simulink model "Scenario_3_v2"  (R2020b)
settings: Solver=ode1be  StartTime=0.0  StopTime=0.5  FixedStep=Ts  MaxStep=Ts/10  MinStep=Ts/40  RelTol=1e-3
values from neighbouring files (symbols this model uses):
  c0 = c0_zeb    (= 6.57988e-09)    [Scenario_17_parameters_v2.m]    (also in Scenario_1_parameters_v2.m; Scenario_2_parameters_v2.m; Scenario_3_parameters_v2.m)
  c0_hawk = 6.37282e-09    [Scenario_17_parameters_v2.m]    (also in Scenario_1_parameters_v2.m; Scenario_2_parameters_v2.m; Scenario_3_parameters_v2.m)
  c1 = c1_zeb    (= 9.15905e-09)    [Scenario_17_parameters_v2.m]    (also in Scenario_1_parameters_v2.m; Scenario_2_parameters_v2.m; Scenario_3_parameters_v2.m)
  c1_hawk = 8.76156e-09    [Scenario_17_parameters_v2.m]    (also in Scenario_1_parameters_v2.m; Scenario_2_parameters_v2.m; Scenario_3_parameters_v2.m)
  fg = 50    [Scenario_17_parameters_v2.m]    (also in Scenario_1_parameters_v2.m; Scenario_2_parameters_v2.m; Scenario_3_parameters_v2.m)
  G10gen = 0.90    (= 0.9)    [Scenario_3_parameters_v2.m]
  G12gen = 0.85    [Scenario_3_parameters_v2.m]
  G1gen = 0.4692    [Scenario_17_parameters_v2.m]    (also in Scenario_1_parameters_v2.m = 0.1; Scenario_2_parameters_v2.m = 0.298581; Scenario_3_parameters_v2.m = 0.65)
  G2gen = 0.80    (= 0.8)    [Scenario_1_parameters_v2.m]    (also in Scenario_2_parameters_v2.m = 0.7; Scenario_3_parameters_v2.m = 0.4)
  G3gen = 0.85    [Scenario_1_parameters_v2.m]    (also in Scenario_2_parameters_v2.m = 0.9; Scenario_3_parameters_v2.m = 0.6)
  G4gen = 0.65    [Scenario_3_parameters_v2.m]
  G5gen = 0.75    [Scenario_17_parameters_v2.m]    (also in Scenario_1_parameters_v2.m = 0.8; Scenario_2_parameters_v2.m = 0.8; Scenario_3_parameters_v2.m = 0.705)
  G6gen = 0.90    (= 0.9)    [Scenario_17_parameters_v2.m]    (also in Scenario_1_parameters_v2.m; Scenario_2_parameters_v2.m = 0.81797; Scenario_3_parameters_v2.m = 0.45)
  G7gen = 0.20    (= 0.2)    [Scenario_17_parameters_v2.m]    (also in Scenario_1_parameters_v2.m = 0.5227; Scenario_2_parameters_v2.m = 0.5098; Scenario_3_parameters_v2.m = 0.4)
  G8gen = 0.58    [Scenario_17_parameters_v2.m]    (also in Scenario_3_parameters_v2.m = 0.65)
  G9gen = 0.8833    [Scenario_17_parameters_v2.m]    (also in Scenario_3_parameters_v2.m = 0.9)
  Iovc = 1.2    [Scenario_17_parameters_v2.m]    (also in Scenario_1_parameters_v2.m; Scenario_2_parameters_v2.m; Scenario_3_parameters_v2.m)
  l0 = l0_zeb    (= 0.00368)    [Scenario_17_parameters_v2.m]    (also in Scenario_1_parameters_v2.m; Scenario_2_parameters_v2.m; Scenario_3_parameters_v2.m)
  l0_hawk = 0.00373    [Scenario_17_parameters_v2.m]    (also in Scenario_1_parameters_v2.m; Scenario_2_parameters_v2.m; Scenario_3_parameters_v2.m)
  l1 = l1_zeb    (= 0.00128)    [Scenario_17_parameters_v2.m]    (also in Scenario_1_parameters_v2.m; Scenario_2_parameters_v2.m; Scenario_3_parameters_v2.m)
  L10dem = 0.04    [Scenario_3_parameters_v2.m]
  L12dem = 0.01    [Scenario_17_parameters_v2.m]    (also in Scenario_3_parameters_v2.m = 0.02)
  L13dem = 0.01    [Scenario_3_parameters_v2.m]
  l1_hawk = 0.00133    [Scenario_17_parameters_v2.m]    (also in Scenario_1_parameters_v2.m; Scenario_2_parameters_v2.m; Scenario_3_parameters_v2.m)
  L1dem = 0.25    [Scenario_17_parameters_v2.m]    (also in Scenario_3_parameters_v2.m = 0.1)
  L3dem = 0.30    (= 0.3)    [Scenario_17_parameters_v2.m]    (also in Scenario_1_parameters_v2.m = 0.1; Scenario_2_parameters_v2.m = 0.1; Scenario_3_parameters_v2.m = 0.2)
  L5dem = 0.25    [Scenario_17_parameters_v2.m]    (also in Scenario_1_parameters_v2.m = 0.35; Scenario_2_parameters_v2.m = 0.35; Scenario_3_parameters_v2.m = 0.1)
  L6dem = 0.15    [Scenario_1_parameters_v2.m]    (also in Scenario_2_parameters_v2.m; Scenario_3_parameters_v2.m = 0.1)
  L7dem = 0.10    (= 0.1)    [Scenario_1_parameters_v2.m]    (also in Scenario_2_parameters_v2.m; Scenario_3_parameters_v2.m = 0.2)
  L9dem = 0.15    [Scenario_17_parameters_v2.m]    (also in Scenario_3_parameters_v2.m = 0.1)
  Pr = Sr*PF    (= 1600500000)    [Scenario_17_parameters_v2.m]    (also in Scenario_1_parameters_v2.m = 1472500000; Scenario_2_parameters_v2.m = 1805000000; Scenario_3_parameters_v2.m = 12740000000)
  Qr = sqrt(Sr^2 - Pr^2)    [Scenario_17_parameters_v2.m]    (also in Scenario_1_parameters_v2.m; Scenario_2_parameters_v2.m; Scenario_3_parameters_v2.m)
  r0 = r0_zeb    (= 0.39362)    [Scenario_17_parameters_v2.m]    (also in Scenario_1_parameters_v2.m; Scenario_2_parameters_v2.m; Scenario_3_parameters_v2.m)
  r0_hawk = 0.44587    [Scenario_17_parameters_v2.m]    (also in Scenario_1_parameters_v2.m; Scenario_2_parameters_v2.m; Scenario_3_parameters_v2.m)
  r1 = r1_zeb    (= 0.06862)    [Scenario_17_parameters_v2.m]    (also in Scenario_1_parameters_v2.m; Scenario_2_parameters_v2.m; Scenario_3_parameters_v2.m)
  r1_hawk = 0.12087    [Scenario_17_parameters_v2.m]    (also in Scenario_1_parameters_v2.m; Scenario_2_parameters_v2.m; Scenario_3_parameters_v2.m)
  Rtpu = Xtpu/40    (= 0.0025)    [Scenario_17_parameters_v2.m]    (also in Scenario_1_parameters_v2.m = 0.00375; Scenario_2_parameters_v2.m = 0.00375; Scenario_3_parameters_v2.m)
  S10non = 500e6    (= 500000000)    [Scenario_3_parameters_v2.m]
  S12non = 250e6    (= 250000000)    [Scenario_3_parameters_v2.m]
  S1non = 700e6    (= 700000000)    [Scenario_17_parameters_v2.m]    (also in Scenario_1_parameters_v2.m = 400000000; Scenario_2_parameters_v2.m = 400000000; Scenario_3_parameters_v2.m = 1000000000)
  S2non = 300e6    (= 300000000)    [Scenario_1_parameters_v2.m]    (also in Scenario_2_parameters_v2.m; Scenario_3_parameters_v2.m = 3000000000)
  S3non = 200e6    (= 200000000)    [Scenario_1_parameters_v2.m]    (also in Scenario_2_parameters_v2.m; Scenario_3_parameters_v2.m = 1000000000)
  S4non = 2000e6    (= 2000000000)    [Scenario_3_parameters_v2.m]
  S5non = 400e6    (= 400000000)    [Scenario_17_parameters_v2.m]    (also in Scenario_1_parameters_v2.m = 500000000; Scenario_2_parameters_v2.m = 500000000; Scenario_3_parameters_v2.m = 2000000000)
  S6non = 150e6    (= 150000000)    [Scenario_17_parameters_v2.m]    (also in Scenario_1_parameters_v2.m = 400000000; Scenario_2_parameters_v2.m = 400000000; Scenario_3_parameters_v2.m = 3000000000)
  S7non = 1500e6    (= 1500000000)    [Scenario_17_parameters_v2.m]    (also in Scenario_1_parameters_v2.m = 200000000; Scenario_2_parameters_v2.m = 200000000; Scenario_3_parameters_v2.m = 4000000000)
  S8non = 600e6    (= 600000000)    [Scenario_17_parameters_v2.m]    (also in Scenario_3_parameters_v2.m = 2000000000)
  S9non = 200e6    (= 200000000)    [Scenario_17_parameters_v2.m]    (also in Scenario_3_parameters_v2.m = 1500000000)
  tonvsc = 0    [Scenario_17_parameters_v2.m]    (also in Scenario_1_parameters_v2.m; Scenario_2_parameters_v2.m; Scenario_3_parameters_v2.m = 0.0001)
  Ts = 50e-6    (= 5e-05)    [Scenario_17_parameters_v2.m]    (also in Scenario_1_parameters_v2.m = 0.0002; Scenario_2_parameters_v2.m = 2e-05; Scenario_3_parameters_v2.m = 0.0001)
  Vhv = 220e3    (= 220000)    [Scenario_17_parameters_v2.m]    (also in Scenario_1_parameters_v2.m; Scenario_2_parameters_v2.m; Scenario_3_parameters_v2.m)
  Vmv = 22e3    (= 22000)    [Scenario_17_parameters_v2.m]    (also in Scenario_1_parameters_v2.m; Scenario_2_parameters_v2.m; Scenario_3_parameters_v2.m)
  w_pll = 2*pi*80    (= 502.654824574)    [Scenario_17_parameters_v2.m]    (also in Scenario_1_parameters_v2.m; Scenario_2_parameters_v2.m; Scenario_3_parameters_v2.m)
  wc1 = wsw1/10    (= 848.230016469)    [Scenario_17_parameters_v2.m]    (also in Scenario_1_parameters_v2.m; Scenario_2_parameters_v2.m; Scenario_3_parameters_v2.m)
  wdc1 = wc1/10    (= 84.8230016469)    [Scenario_17_parameters_v2.m]    (also in Scenario_1_parameters_v2.m; Scenario_2_parameters_v2.m; Scenario_3_parameters_v2.m)
  wpq1 = wc1/10    (= 84.8230016469)    [Scenario_17_parameters_v2.m]    (also in Scenario_1_parameters_v2.m; Scenario_2_parameters_v2.m; Scenario_3_parameters_v2.m)
  wsw1 = ksw1*2*pi*fg    (= 8482.30016469)    [Scenario_17_parameters_v2.m]    (also in Scenario_1_parameters_v2.m; Scenario_2_parameters_v2.m; Scenario_3_parameters_v2.m)
  Xtpu = 0.10    (= 0.1)    [Scenario_17_parameters_v2.m]    (also in Scenario_1_parameters_v2.m = 0.15; Scenario_2_parameters_v2.m = 0.15; Scenario_3_parameters_v2.m)
undefined symbols (not defined in the file or in its folder): D11, Delta
libraries: powerlib x428, simulink_extras x272, powerlib_meascontrol x194, pid_lib x105, simulink x60, eeTransforms x54, spsFirstOrderFilterLib x36, eePwmGeneratorTwoLevel x9
(part 8 of 40)

== system Scenario_3_v2/G6/VSC v2 ==
  note: If using different transformer connection,
      | compensate the delay in the modulation
  Pset : Inport
  Qset : Inport  Port=2
  Block : Step  Time=tonvsc  Before=1  After=0  SampleTime=0
  NOT : Logic  Operator=NOT  IconShape=distinctive  AllPortsSameDT=off  OutDataTypeStr=boolean
  Three-Phase Transformer (Two Windings) : powerlib/Elements/Three-Phase Transformer (Two Windings)  Winding1Connection=Yg  Winding2Connection=Delta (D11)  CoreType=Three single-phase transformers  SetSaturation=off  Hysteresis=off  DataFile='hysteresis'  SetInitialFlux=off  Measurements=None  UNITS=pu  NominalPower=[Pconv , fg ]  Winding1=[Vhv, Rtpu/2, Xtpu/2]  Winding2=[Vmv, Rtpu/2, Xtpu/2]  Rm=5000  Lm=5000  L0=0.5  Saturation=[ 0,0 ; 0.0024,1.2 ; 1.0,1.52 ]  InitialFluxes=[ 0.8 , -0.8 , 0.7 ]  BreakLoop=off  DiscreteSolver=Trapezoidal iterative  DataType=off  TransfoNumber=1
  Three-Phase Breaker : powerlib/Elements/Three-Phase Breaker  InitialState=open  SwitchA=on  SwitchB=on  SwitchC=on  SwitchTimes="[1/60  5/60]"  External=on  BreakerResistance=0.001  SnubberResistance=1e7  SnubberCapacitance=inf  Measurements=None
  VI measurement : Subsystem
      settings: PortSchema="{\"entries\":[{\"content\":{\"sides\":[{\"content\":{\"connectorIds\":[\"LConn1\",\"LConn2\",\"LConn3\"]},\"type\":\"ConnectorPlacement.EquallySpacedRectSide\",\"uuid\":\"d0d5b0b8-afec-4f90-9eba-536a06b10059\"},{\"content\":{\"connectorIds\":[\"RConn1\",\"RConn2\",\"RConn3\"],\"side\":\"RIGHT\"},\"type\":\"ConnectorPlacement.EquallySpacedRectSide\",\"uuid\":\"adc1b68d-6172-4507-b54b-9373921355a1\"},{\"content\":{\"connectorIds\":[\"Out1\",\"Out2\"],\"side\":\"TOP\"},\"type\":\"ConnectorPlacement.EquallySpacedRectSide\",\"uuid\":\"8c5adf07-e95b-4907-94c3-1b2a47d47f40\"}]},\"type\":\"ConnectorPlacement.EquallySpacedConnector\",\"uuid\":\"87d0b20f-8f85-4790-a611-3415e642a83a\"}],\"packageUris\":[\"http://schema.mathworks.com/mf0/Connector/R2020b\"],\"version\":\"1.0\"}"
  VSC Control : Subsystem
      settings: PortSchema="{\"entries\":[{\"content\":{\"sides\":[{\"content\":{\"connectorIds\":[\"In1\",\"In2\",\"In3\",\"In4\",\"In5\",\"In6\"]},\"type\":\"ConnectorPlacement.EquallySpacedRectSide\",\"uuid\":\"cada8d9e-53e0-4197-9386-6c7b6ea13844\"},{\"content\":{\"connectorIds\":[\"Out1\"],\"side\":\"RIGHT\"},\"type\":\"ConnectorPlacement.EquallySpacedRectSide\",\"uuid\":\"f237b52a-0d77-45c0-937d-32cafba1283e\"},{\"content\":{\"connectorIds\":[\"Out2\"],\"side\":\"TOP\"},\"type\":\"ConnectorPlacement.EquallySpacedRectSide\",\"uuid\":\"e6f268b5-5f09-49a6-9529-b1aeebd5f021\"}]},\"type\":\"ConnectorPlacement.EquallySpacedConnector\",\"uuid\":\"4d1d2957-2eb9-4111-8c87-957e800b2b0b\"}],\"packageUris\":[\"http://schema.mathworks.com/mf0/Connector/R2020b\"],\"version\":\"1.0\"}"
  VSC Model : Subsystem  Variant=on  VariantControlMode=label  LabelModeActiveChoice=EMT_AVG
      settings: PortSchema="{\"entries\":[{\"content\":{\"sides\":[{\"content\":{\"connectorIds\":[\"LConn1\",\"LConn2\",\"LConn3\"]},\"type\":\"ConnectorPlacement.EquallySpacedRectSide\",\"uuid\":\"96043b84-a665-4cb2-a938-d6633d7ee474\"},{\"content\":{\"connectorIds\":[\"In1\"],\"side\":\"RIGHT\"},\"type\":\"ConnectorPlacement.EquallySpacedRectSide\",\"uuid\":\"064d463f-c23a-42ac-89ce-8dea3d446214\"},{\"content\":{\"connectorIds\":[],\"side\":\"TOP\"},\"type\":\"ConnectorPlacement.EquallySpacedRectSide\",\"uuid\":\"95ef669c-c6ed-44c3-8b69-447906728b6d\"}]},\"type\":\"ConnectorPlacement.EquallySpacedConnector\",\"uuid\":\"ea66db09-64d7-4d7e-ba7b-d769c56e2dbd\"}],\"packageUris\":[\"http://schema.mathworks.com/mf0/Connector/19700101\"],\"version\":\"1.0\"}"
  output signals : Subsystem
  A : PMIOPort  Side=Left
  B : PMIOPort  Port=2  Side=Left
  C : PMIOPort  Port=3  Side=Left
  m : Outport
  wires:
  NOT/1 -> Three-Phase Breaker/1
  VSC Control/1(Ref) -> VSC Model/1(Ref)
  [Is] -> VSC Control/3(Iabc)
  Block/1 -> NOT/1, VSC Control/1(Block)
  [Vs] -> output signals/1(Vs)
  [Is] -> output signals/2(Is)
  VSC Control/2(m) -> output signals/3(control)
  output signals/1(m) -> m/1
  VI measurement/1(Vs) -> [Vs]
  VI measurement/2(Is) -> [Is]
  Qset/1 -> VSC Control/5(Qset)
  [Vs] -> VSC Control/2(Vabc)
  ? -> VSC Control/6(Edc)
  Pset/1 -> VSC Control/4(Pset)
  connections:
  Three-Phase Transformer (Two Windings)/LConn3 -- Three-Phase Breaker/LConn3
  Three-Phase Transformer (Two Windings)/LConn2 -- Three-Phase Breaker/LConn2
  Three-Phase Transformer (Two Windings)/LConn1 -- Three-Phase Breaker/LConn1
  Three-Phase Transformer (Two Windings)/RConn3 -- VSC Model/LConn3
  Three-Phase Transformer (Two Windings)/RConn2 -- VSC Model/LConn2
  Three-Phase Transformer (Two Windings)/RConn1 -- VSC Model/LConn1
  VI measurement/RConn1 -- A/RConn1
  VI measurement/RConn2 -- B/RConn1
  VI measurement/RConn3 -- C/RConn1
  VI measurement/LConn1 -- Three-Phase Breaker/RConn1
  VI measurement/LConn2 -- Three-Phase Breaker/RConn2
  VI measurement/LConn3 -- Three-Phase Breaker/RConn3

== system Scenario_3_v2/G7/VSC v2 ==
  note: If using different transformer connection,
      | compensate the delay in the modulation
  Pset : Inport
  Qset : Inport  Port=2
  Block : Step  Time=tonvsc  Before=1  After=0  SampleTime=0
  NOT : Logic  Operator=NOT  IconShape=distinctive  AllPortsSameDT=off  OutDataTypeStr=boolean
  Three-Phase Transformer (Two Windings) : powerlib/Elements/Three-Phase Transformer (Two Windings)  Winding1Connection=Yg  Winding2Connection=Delta (D11)  CoreType=Three single-phase transformers  SetSaturation=off  Hysteresis=off  DataFile='hysteresis'  SetInitialFlux=off  Measurements=None  UNITS=pu  NominalPower=[Pconv , fg ]  Winding1=[Vhv, Rtpu/2, Xtpu/2]  Winding2=[Vmv, Rtpu/2, Xtpu/2]  Rm=5000  Lm=5000  L0=0.5  Saturation=[ 0,0 ; 0.0024,1.2 ; 1.0,1.52 ]  InitialFluxes=[ 0.8 , -0.8 , 0.7 ]  BreakLoop=off  DiscreteSolver=Trapezoidal iterative  DataType=off  TransfoNumber=1
  Three-Phase Breaker : powerlib/Elements/Three-Phase Breaker  InitialState=open  SwitchA=on  SwitchB=on  SwitchC=on  SwitchTimes="[1/60  5/60]"  External=on  BreakerResistance=0.001  SnubberResistance=1e7  SnubberCapacitance=inf  Measurements=None
  VI measurement : Subsystem
      settings: PortSchema="{\"entries\":[{\"content\":{\"sides\":[{\"content\":{\"connectorIds\":[\"LConn1\",\"LConn2\",\"LConn3\"]},\"type\":\"ConnectorPlacement.EquallySpacedRectSide\",\"uuid\":\"d0d5b0b8-afec-4f90-9eba-536a06b10059\"},{\"content\":{\"connectorIds\":[\"RConn1\",\"RConn2\",\"RConn3\"],\"side\":\"RIGHT\"},\"type\":\"ConnectorPlacement.EquallySpacedRectSide\",\"uuid\":\"adc1b68d-6172-4507-b54b-9373921355a1\"},{\"content\":{\"connectorIds\":[\"Out1\",\"Out2\"],\"side\":\"TOP\"},\"type\":\"ConnectorPlacement.EquallySpacedRectSide\",\"uuid\":\"8c5adf07-e95b-4907-94c3-1b2a47d47f40\"}]},\"type\":\"ConnectorPlacement.EquallySpacedConnector\",\"uuid\":\"87d0b20f-8f85-4790-a611-3415e642a83a\"}],\"packageUris\":[\"http://schema.mathworks.com/mf0/Connector/R2020b\"],\"version\":\"1.0\"}"
  VSC Control : Subsystem
      settings: PortSchema="{\"entries\":[{\"content\":{\"sides\":[{\"content\":{\"connectorIds\":[\"In1\",\"In2\",\"In3\",\"In4\",\"In5\",\"In6\"]},\"type\":\"ConnectorPlacement.EquallySpacedRectSide\",\"uuid\":\"cada8d9e-53e0-4197-9386-6c7b6ea13844\"},{\"content\":{\"connectorIds\":[\"Out1\"],\"side\":\"RIGHT\"},\"type\":\"ConnectorPlacement.EquallySpacedRectSide\",\"uuid\":\"f237b52a-0d77-45c0-937d-32cafba1283e\"},{\"content\":{\"connectorIds\":[\"Out2\"],\"side\":\"TOP\"},\"type\":\"ConnectorPlacement.EquallySpacedRectSide\",\"uuid\":\"e6f268b5-5f09-49a6-9529-b1aeebd5f021\"}]},\"type\":\"ConnectorPlacement.EquallySpacedConnector\",\"uuid\":\"4d1d2957-2eb9-4111-8c87-957e800b2b0b\"}],\"packageUris\":[\"http://schema.mathworks.com/mf0/Connector/R2020b\"],\"version\":\"1.0\"}"
  VSC Model : Subsystem  Variant=on  VariantControlMode=label  LabelModeActiveChoice=EMT_AVG
      settings: PortSchema="{\"entries\":[{\"content\":{\"sides\":[{\"content\":{\"connectorIds\":[\"LConn1\",\"LConn2\",\"LConn3\"]},\"type\":\"ConnectorPlacement.EquallySpacedRectSide\",\"uuid\":\"96043b84-a665-4cb2-a938-d6633d7ee474\"},{\"content\":{\"connectorIds\":[\"In1\"],\"side\":\"RIGHT\"},\"type\":\"ConnectorPlacement.EquallySpacedRectSide\",\"uuid\":\"064d463f-c23a-42ac-89ce-8dea3d446214\"},{\"content\":{\"connectorIds\":[],\"side\":\"TOP\"},\"type\":\"ConnectorPlacement.EquallySpacedRectSide\",\"uuid\":\"95ef669c-c6ed-44c3-8b69-447906728b6d\"}]},\"type\":\"ConnectorPlacement.EquallySpacedConnector\",\"uuid\":\"ea66db09-64d7-4d7e-ba7b-d769c56e2dbd\"}],\"packageUris\":[\"http://schema.mathworks.com/mf0/Connector/19700101\"],\"version\":\"1.0\"}"
  output signals : Subsystem
  A : PMIOPort  Side=Left
  B : PMIOPort  Port=2  Side=Left
  C : PMIOPort  Port=3  Side=Left
  m : Outport
  wires:
  NOT/1 -> Three-Phase Breaker/1
  VSC Control/1(Ref) -> VSC Model/1(Ref)
  [Is] -> VSC Control/3(Iabc)
  Block/1 -> NOT/1, VSC Control/1(Block)
  [Vs] -> output signals/1(Vs)
  [Is] -> output signals/2(Is)
  VSC Control/2(m) -> output signals/3(control)
  output signals/1(m) -> m/1
  VI measurement/1(Vs) -> [Vs]
  VI measurement/2(Is) -> [Is]
  Qset/1 -> VSC Control/5(Qset)
  [Vs] -> VSC Control/2(Vabc)
  ? -> VSC Control/6(Edc)
  Pset/1 -> VSC Control/4(Pset)
  connections:
  Three-Phase Transformer (Two Windings)/LConn3 -- Three-Phase Breaker/LConn3
  Three-Phase Transformer (Two Windings)/LConn2 -- Three-Phase Breaker/LConn2
  Three-Phase Transformer (Two Windings)/LConn1 -- Three-Phase Breaker/LConn1
  Three-Phase Transformer (Two Windings)/RConn3 -- VSC Model/LConn3
  Three-Phase Transformer (Two Windings)/RConn2 -- VSC Model/LConn2
  Three-Phase Transformer (Two Windings)/RConn1 -- VSC Model/LConn1
  VI measurement/RConn1 -- A/RConn1
  VI measurement/RConn2 -- B/RConn1
  VI measurement/RConn3 -- C/RConn1
  VI measurement/LConn1 -- Three-Phase Breaker/RConn1
  VI measurement/LConn2 -- Three-Phase Breaker/RConn2
  VI measurement/LConn3 -- Three-Phase Breaker/RConn3

== system Scenario_3_v2/G9/VSC v2 ==
  note: If using different transformer connection,
      | compensate the delay in the modulation
  Pset : Inport
  Qset : Inport  Port=2
  Block : Step  Time=tonvsc  Before=1  After=0  SampleTime=0
  NOT : Logic  Operator=NOT  IconShape=distinctive  AllPortsSameDT=off  OutDataTypeStr=boolean
  Three-Phase Transformer (Two Windings) : powerlib/Elements/Three-Phase Transformer (Two Windings)  Winding1Connection=Yg  Winding2Connection=Delta (D11)  CoreType=Three single-phase transformers  SetSaturation=off  Hysteresis=off  DataFile='hysteresis'  SetInitialFlux=off  Measurements=None  UNITS=pu  NominalPower=[Pconv , fg ]  Winding1=[Vhv, Rtpu/2, Xtpu/2]  Winding2=[Vmv, Rtpu/2, Xtpu/2]  Rm=5000  Lm=5000  L0=0.5  Saturation=[ 0,0 ; 0.0024,1.2 ; 1.0,1.52 ]  InitialFluxes=[ 0.8 , -0.8 , 0.7 ]  BreakLoop=off  DiscreteSolver=Trapezoidal iterative  DataType=off  TransfoNumber=1
  Three-Phase Breaker : powerlib/Elements/Three-Phase Breaker  InitialState=open  SwitchA=on  SwitchB=on  SwitchC=on  SwitchTimes="[1/60  5/60]"  External=on  BreakerResistance=0.001  SnubberResistance=1e7  SnubberCapacitance=inf  Measurements=None
  VI measurement : Subsystem
      settings: PortSchema="{\"entries\":[{\"content\":{\"sides\":[{\"content\":{\"connectorIds\":[\"LConn1\",\"LConn2\",\"LConn3\"]},\"type\":\"ConnectorPlacement.EquallySpacedRectSide\",\"uuid\":\"d0d5b0b8-afec-4f90-9eba-536a06b10059\"},{\"content\":{\"connectorIds\":[\"RConn1\",\"RConn2\",\"RConn3\"],\"side\":\"RIGHT\"},\"type\":\"ConnectorPlacement.EquallySpacedRectSide\",\"uuid\":\"adc1b68d-6172-4507-b54b-9373921355a1\"},{\"content\":{\"connectorIds\":[\"Out1\",\"Out2\"],\"side\":\"TOP\"},\"type\":\"ConnectorPlacement.EquallySpacedRectSide\",\"uuid\":\"8c5adf07-e95b-4907-94c3-1b2a47d47f40\"}]},\"type\":\"ConnectorPlacement.EquallySpacedConnector\",\"uuid\":\"87d0b20f-8f85-4790-a611-3415e642a83a\"}],\"packageUris\":[\"http://schema.mathworks.com/mf0/Connector/R2020b\"],\"version\":\"1.0\"}"
  VSC Control : Subsystem
      settings: PortSchema="{\"entries\":[{\"content\":{\"sides\":[{\"content\":{\"connectorIds\":[\"In1\",\"In2\",\"In3\",\"In4\",\"In5\",\"In6\"]},\"type\":\"ConnectorPlacement.EquallySpacedRectSide\",\"uuid\":\"cada8d9e-53e0-4197-9386-6c7b6ea13844\"},{\"content\":{\"connectorIds\":[\"Out1\"],\"side\":\"RIGHT\"},\"type\":\"ConnectorPlacement.EquallySpacedRectSide\",\"uuid\":\"f237b52a-0d77-45c0-937d-32cafba1283e\"},{\"content\":{\"connectorIds\":[\"Out2\"],\"side\":\"TOP\"},\"type\":\"ConnectorPlacement.EquallySpacedRectSide\",\"uuid\":\"e6f268b5-5f09-49a6-9529-b1aeebd5f021\"}]},\"type\":\"ConnectorPlacement.EquallySpacedConnector\",\"uuid\":\"4d1d2957-2eb9-4111-8c87-957e800b2b0b\"}],\"packageUris\":[\"http://schema.mathworks.com/mf0/Connector/R2020b\"],\"version\":\"1.0\"}"
  VSC Model : Subsystem  Variant=on  VariantControlMode=label  LabelModeActiveChoice=EMT_AVG
      settings: PortSchema="{\"entries\":[{\"content\":{\"sides\":[{\"content\":{\"connectorIds\":[\"LConn1\",\"LConn2\",\"LConn3\"]},\"type\":\"ConnectorPlacement.EquallySpacedRectSide\",\"uuid\":\"96043b84-a665-4cb2-a938-d6633d7ee474\"},{\"content\":{\"connectorIds\":[\"In1\"],\"side\":\"RIGHT\"},\"type\":\"ConnectorPlacement.EquallySpacedRectSide\",\"uuid\":\"064d463f-c23a-42ac-89ce-8dea3d446214\"},{\"content\":{\"connectorIds\":[],\"side\":\"TOP\"},\"type\":\"ConnectorPlacement.EquallySpacedRectSide\",\"uuid\":\"95ef669c-c6ed-44c3-8b69-447906728b6d\"}]},\"type\":\"ConnectorPlacement.EquallySpacedConnector\",\"uuid\":\"ea66db09-64d7-4d7e-ba7b-d769c56e2dbd\"}],\"packageUris\":[\"http://schema.mathworks.com/mf0/Connector/19700101\"],\"version\":\"1.0\"}"
  output signals : Subsystem
  A : PMIOPort  Side=Left
  B : PMIOPort  Port=2  Side=Left
  C : PMIOPort  Port=3  Side=Left
  m : Outport
  wires:
  NOT/1 -> Three-Phase Breaker/1
  VSC Control/1(Ref) -> VSC Model/1(Ref)
  [Is] -> VSC Control/3(Iabc)
  Block/1 -> NOT/1, VSC Control/1(Block)
  [Vs] -> output signals/1(Vs)
  [Is] -> output signals/2(Is)
  VSC Control/2(m) -> output signals/3(control)
  output signals/1(m) -> m/1
  VI measurement/1(Vs) -> [Vs]
  VI measurement/2(Is) -> [Is]
  Qset/1 -> VSC Control/5(Qset)
  [Vs] -> VSC Control/2(Vabc)
  ? -> VSC Control/6(Edc)
  Pset/1 -> VSC Control/4(Pset)
  connections:
  Three-Phase Transformer (Two Windings)/LConn3 -- Three-Phase Breaker/LConn3
  Three-Phase Transformer (Two Windings)/LConn2 -- Three-Phase Breaker/LConn2
  Three-Phase Transformer (Two Windings)/LConn1 -- Three-Phase Breaker/LConn1
  Three-Phase Transformer (Two Windings)/RConn3 -- VSC Model/LConn3
  Three-Phase Transformer (Two Windings)/RConn2 -- VSC Model/LConn2
  Three-Phase Transformer (Two Windings)/RConn1 -- VSC Model/LConn1
  VI measurement/RConn1 -- A/RConn1
  VI measurement/RConn2 -- B/RConn1
  VI measurement/RConn3 -- C/RConn1
  VI measurement/LConn1 -- Three-Phase Breaker/RConn1
  VI measurement/LConn2 -- Three-Phase Breaker/RConn2
  VI measurement/LConn3 -- Three-Phase Breaker/RConn3

== system Scenario_3_v2/HVDC/DC-link ==
  note: Diagram of the DC link
  note: The DC link dynamics is calculated in state-space intead of simulated using electric elements to allow both EMT and Phasor use the same block in the simulations
  note: | vdc1 |
      | x = | vdc2 |
      | | idc |
  note: The model states are the DC voltages of the two terminals and the DC current:
  note: idc1
  note: idc2
  note: The model outputs are the DC voltages of the two terminals
  idc1 : Inport
  idc2 : Inport  Port=2
  C1 : powerlib/Elements/Series RLC Branch  Commented=on  LConnTagsString=__new0  RConnTagsString=__new0  BranchType=C  Resistance=R  Inductance=1e-3  SetiL0=off  InitialCurrent=0  Capacitance=1  Setx0=off  InitialVoltage=Vdc0  Measurements=None
  C2 : powerlib/Elements/Series RLC Branch  Commented=on  LConnTagsString=__new0  RConnTagsString=__new0  BranchType=C  Resistance=R  Inductance=1e-3  SetiL0=off  InitialCurrent=0  Capacitance=1  Setx0=off  InitialVoltage=Vdc0  Measurements=None
  Demux : Demux  Outputs=2
  Mux : Mux  Inputs=2
  RL : powerlib/Elements/Series RLC Branch  Commented=on  LConnTagsString=__new0  RConnTagsString=__new0  BranchType=RL  Resistance=1  Inductance=1  SetiL0=off  InitialCurrent=0  Capacitance=1e-6  Setx0=off  InitialVoltage=0  Measurements=None
  State-Space1 : StateSpace  A=[0 0 -1/C1 ; 0 0 1/C2 ; 1/L -1/L -R/L]  B=[1/C1 0 ; 0 1/C2; 0 0]  C=[1 0 0; 0 1 0]  D=[0 0; 0 0]  InitialCondition=[v1dc0; v2dc0; idc0]
  vdc1 : Outport
  vdc2 : Outport  Port=2
  wires:
  ? -> ?
  ? -> ?
  Mux/1 -> State-Space1/1
  idc1/1 -> Mux/1
  idc2/1 -> Mux/2
  State-Space1/1 -> Demux/1
  Demux/1 -> vdc1/1
  Demux/2 -> vdc2/1
  connections:
  C1/LConn1 -- RL/LConn1
  C2/LConn1 -- RL/RConn1

== system Scenario_3_v2/HVDC/VSC1 v2 ==
  note: If using different transformer connection,
      | compensate the delay in the modulation
  Pset : Inport
  Qset : Inport  Port=2
  Block : Step  Time=tonvsc  Before=1  After=0  SampleTime=0
  NOT : Logic  Operator=NOT  IconShape=distinctive  AllPortsSameDT=off  OutDataTypeStr=boolean
  Three-Phase Transformer (Two Windings) : powerlib/Elements/Three-Phase Transformer (Two Windings)  Winding1Connection=Yg  Winding2Connection=Delta (D11)  CoreType=Three single-phase transformers  SetSaturation=off  Hysteresis=off  DataFile='hysteresis'  SetInitialFlux=off  Measurements=None  UNITS=pu  NominalPower=[Pconv , fg ]  Winding1=[Vhv, Rtpu/2, Xtpu/2]  Winding2=[Vmv, Rtpu/2, Xtpu/2]  Rm=5000  Lm=5000  L0=0.5  Saturation=[ 0,0 ; 0.0024,1.2 ; 1.0,1.52 ]  InitialFluxes=[ 0.8 , -0.8 , 0.7 ]  BreakLoop=off  DiscreteSolver=Trapezoidal iterative  DataType=off  TransfoNumber=1
  Three-Phase Breaker : powerlib/Elements/Three-Phase Breaker  InitialState=open  SwitchA=on  SwitchB=on  SwitchC=on  SwitchTimes="[1/60  5/60]"  External=on  BreakerResistance=0.001  SnubberResistance=1e7  SnubberCapacitance=inf  Measurements=None
  VI measurement : Subsystem
      settings: PortSchema="{\"entries\":[{\"content\":{\"sides\":[{\"content\":{\"connectorIds\":[\"LConn1\",\"LConn2\",\"LConn3\"]},\"type\":\"ConnectorPlacement.EquallySpacedRectSide\",\"uuid\":\"d0d5b0b8-afec-4f90-9eba-536a06b10059\"},{\"content\":{\"connectorIds\":[\"RConn1\",\"RConn2\",\"RConn3\"],\"side\":\"RIGHT\"},\"type\":\"ConnectorPlacement.EquallySpacedRectSide\",\"uuid\":\"adc1b68d-6172-4507-b54b-9373921355a1\"},{\"content\":{\"connectorIds\":[\"Out1\",\"Out2\"],\"side\":\"TOP\"},\"type\":\"ConnectorPlacement.EquallySpacedRectSide\",\"uuid\":\"8c5adf07-e95b-4907-94c3-1b2a47d47f40\"}]},\"type\":\"ConnectorPlacement.EquallySpacedConnector\",\"uuid\":\"87d0b20f-8f85-4790-a611-3415e642a83a\"}],\"packageUris\":[\"http://schema.mathworks.com/mf0/Connector/R2020b\"],\"version\":\"1.0\"}"
  VSC Control : Subsystem
      settings: PortSchema="{\"entries\":[{\"content\":{\"sides\":[{\"content\":{\"connectorIds\":[\"In1\",\"In2\",\"In3\",\"In4\",\"In5\"]},\"type\":\"ConnectorPlacement.EquallySpacedRectSide\",\"uuid\":\"cada8d9e-53e0-4197-9386-6c7b6ea13844\"},{\"content\":{\"connectorIds\":[\"Out1\"],\"side\":\"RIGHT\"},\"type\":\"ConnectorPlacement.EquallySpacedRectSide\",\"uuid\":\"f237b52a-0d77-45c0-937d-32cafba1283e\"},{\"content\":{\"connectorIds\":[\"Out2\"],\"side\":\"TOP\"},\"type\":\"ConnectorPlacement.EquallySpacedRectSide\",\"uuid\":\"e6f268b5-5f09-49a6-9529-b1aeebd5f021\"}]},\"type\":\"ConnectorPlacement.EquallySpacedConnector\",\"uuid\":\"4d1d2957-2eb9-4111-8c87-957e800b2b0b\"}],\"packageUris\":[\"http://schema.mathworks.com/mf0/Connector/19700101\"],\"version\":\"1.0\"}"
  VSC Model : Subsystem  Variant=on  VariantControlMode=label  LabelModeActiveChoice=EMT_AVG
      settings: PortSchema="{\"entries\":[{\"content\":{\"sides\":[{\"content\":{\"connectorIds\":[\"LConn1\",\"LConn2\",\"LConn3\"]},\"type\":\"ConnectorPlacement.EquallySpacedRectSide\",\"uuid\":\"96043b84-a665-4cb2-a938-d6633d7ee474\"},{\"content\":{\"connectorIds\":[\"In1\"],\"side\":\"RIGHT\"},\"type\":\"ConnectorPlacement.EquallySpacedRectSide\",\"uuid\":\"064d463f-c23a-42ac-89ce-8dea3d446214\"},{\"content\":{\"connectorIds\":[],\"side\":\"TOP\"},\"type\":\"ConnectorPlacement.EquallySpacedRectSide\",\"uuid\":\"95ef669c-c6ed-44c3-8b69-447906728b6d\"}]},\"type\":\"ConnectorPlacement.EquallySpacedConnector\",\"uuid\":\"ea66db09-64d7-4d7e-ba7b-d769c56e2dbd\"}],\"packageUris\":[\"http://schema.mathworks.com/mf0/Connector/19700101\"],\"version\":\"1.0\"}"
  output signals : Subsystem
  A : PMIOPort  Side=Left
  B : PMIOPort  Port=2  Side=Left
  C : PMIOPort  Port=3  Side=Left
  m : Outport
  wires:
  NOT/1 -> Three-Phase Breaker/1
  VSC Control/1(Ref) -> VSC Model/1(Ref)
  [Is] -> VSC Control/3(Iabc)
  Block/1 -> NOT/1, VSC Control/1(Block)
  [Vs] -> output signals/1(Vs)
  [Is] -> output signals/2(Is)
  VSC Control/2(m) -> output signals/3(control)
  output signals/1(m) -> m/1
  VI measurement/1(Vs) -> [Vs]
  VI measurement/2(Is) -> [Is]
  Qset/1 -> VSC Control/5(Qset)
  Pset/1 -> VSC Control/4(Pset)
  [Vs] -> VSC Control/2(Vabc)
  connections:
  Three-Phase Transformer (Two Windings)/LConn3 -- Three-Phase Breaker/LConn3
  Three-Phase Transformer (Two Windings)/LConn2 -- Three-Phase Breaker/LConn2
  Three-Phase Transformer (Two Windings)/LConn1 -- Three-Phase Breaker/LConn1
  Three-Phase Transformer (Two Windings)/RConn3 -- VSC Model/LConn3
  Three-Phase Transformer (Two Windings)/RConn2 -- VSC Model/LConn2
  Three-Phase Transformer (Two Windings)/RConn1 -- VSC Model/LConn1
  VI measurement/RConn1 -- A/RConn1
  VI measurement/RConn2 -- B/RConn1
  VI measurement/RConn3 -- C/RConn1
  VI measurement/LConn1 -- Three-Phase Breaker/RConn1
  VI measurement/LConn2 -- Three-Phase Breaker/RConn2
  VI measurement/LConn3 -- Three-Phase Breaker/RConn3

== system Scenario_3_v2/HVDC/VSC2 v2 ==
  note: If using different transformer connection,
      | compensate the delay in the modulation
  Qset : Inport
  Edc : Inport  Port=2
  Block : Step  Time=tonvsc  Before=1  After=0  SampleTime=0
  NOT : Logic  Operator=NOT  IconShape=distinctive  AllPortsSameDT=off  OutDataTypeStr=boolean
  Three-Phase Transformer (Two Windings) : powerlib/Elements/Three-Phase Transformer (Two Windings)  Winding1Connection=Yg  Winding2Connection=Delta (D11)  CoreType=Three single-phase transformers  SetSaturation=off  Hysteresis=off  DataFile='hysteresis'  SetInitialFlux=off  Measurements=None  UNITS=pu  NominalPower=[Pconv , fg ]  Winding1=[Vhv, Rtpu/2, Xtpu/2]  Winding2=[Vmv, Rtpu/2, Xtpu/2]  Rm=5000  Lm=5000  L0=0.5  Saturation=[ 0,0 ; 0.0024,1.2 ; 1.0,1.52 ]  InitialFluxes=[ 0.8 , -0.8 , 0.7 ]  BreakLoop=off  DiscreteSolver=Trapezoidal iterative  DataType=off  TransfoNumber=1
  Three-Phase Breaker : powerlib/Elements/Three-Phase Breaker  InitialState=open  SwitchA=on  SwitchB=on  SwitchC=on  SwitchTimes="[1/60  5/60]"  External=on  BreakerResistance=0.001  SnubberResistance=1e7  SnubberCapacitance=inf  Measurements=None
  VI measurement : Subsystem
      settings: PortSchema="{\"entries\":[{\"content\":{\"sides\":[{\"content\":{\"connectorIds\":[\"LConn1\",\"LConn2\",\"LConn3\"]},\"type\":\"ConnectorPlacement.EquallySpacedRectSide\",\"uuid\":\"d0d5b0b8-afec-4f90-9eba-536a06b10059\"},{\"content\":{\"connectorIds\":[\"RConn1\",\"RConn2\",\"RConn3\"],\"side\":\"RIGHT\"},\"type\":\"ConnectorPlacement.EquallySpacedRectSide\",\"uuid\":\"adc1b68d-6172-4507-b54b-9373921355a1\"},{\"content\":{\"connectorIds\":[\"Out1\",\"Out2\"],\"side\":\"TOP\"},\"type\":\"ConnectorPlacement.EquallySpacedRectSide\",\"uuid\":\"8c5adf07-e95b-4907-94c3-1b2a47d47f40\"}]},\"type\":\"ConnectorPlacement.EquallySpacedConnector\",\"uuid\":\"87d0b20f-8f85-4790-a611-3415e642a83a\"}],\"packageUris\":[\"http://schema.mathworks.com/mf0/Connector/R2020b\"],\"version\":\"1.0\"}"
  VSC Control : Subsystem
      settings: PortSchema="{\"entries\":[{\"content\":{\"sides\":[{\"content\":{\"connectorIds\":[\"In1\",\"In2\",\"In3\",\"In4\",\"In5\",\"In6\"]},\"type\":\"ConnectorPlacement.EquallySpacedRectSide\",\"uuid\":\"cada8d9e-53e0-4197-9386-6c7b6ea13844\"},{\"content\":{\"connectorIds\":[\"Out1\"],\"side\":\"RIGHT\"},\"type\":\"ConnectorPlacement.EquallySpacedRectSide\",\"uuid\":\"f237b52a-0d77-45c0-937d-32cafba1283e\"},{\"content\":{\"connectorIds\":[\"Out2\"],\"side\":\"TOP\"},\"type\":\"ConnectorPlacement.EquallySpacedRectSide\",\"uuid\":\"e6f268b5-5f09-49a6-9529-b1aeebd5f021\"}]},\"type\":\"ConnectorPlacement.EquallySpacedConnector\",\"uuid\":\"4d1d2957-2eb9-4111-8c87-957e800b2b0b\"}],\"packageUris\":[\"http://schema.mathworks.com/mf0/Connector/R2020b\"],\"version\":\"1.0\"}"
  VSC Model : Subsystem  Variant=on  VariantControlMode=label  LabelModeActiveChoice=EMT_AVG
      settings: PortSchema="{\"entries\":[{\"content\":{\"sides\":[{\"content\":{\"connectorIds\":[\"LConn1\",\"LConn2\",\"LConn3\"]},\"type\":\"ConnectorPlacement.EquallySpacedRectSide\",\"uuid\":\"96043b84-a665-4cb2-a938-d6633d7ee474\"},{\"content\":{\"connectorIds\":[\"In1\"],\"side\":\"RIGHT\"},\"type\":\"ConnectorPlacement.EquallySpacedRectSide\",\"uuid\":\"064d463f-c23a-42ac-89ce-8dea3d446214\"},{\"content\":{\"connectorIds\":[],\"side\":\"TOP\"},\"type\":\"ConnectorPlacement.EquallySpacedRectSide\",\"uuid\":\"95ef669c-c6ed-44c3-8b69-447906728b6d\"}]},\"type\":\"ConnectorPlacement.EquallySpacedConnector\",\"uuid\":\"ea66db09-64d7-4d7e-ba7b-d769c56e2dbd\"}],\"packageUris\":[\"http://schema.mathworks.com/mf0/Connector/19700101\"],\"version\":\"1.0\"}"
  output signals : Subsystem
  A : PMIOPort  Side=Left
  B : PMIOPort  Port=2  Side=Left
  C : PMIOPort  Port=3  Side=Left
  m : Outport
  wires:
  NOT/1 -> Three-Phase Breaker/1
  VSC Control/1(Ref) -> VSC Model/1(Ref)
  [Is] -> VSC Control/3(Iabc)
  Block/1 -> NOT/1, VSC Control/1(Block)
  [Vs] -> output signals/1(Vs)
  [Is] -> output signals/2(Is)
  VSC Control/2(m) -> output signals/3(control)
  output signals/1(m) -> m/1
  VI measurement/1(Vs) -> [Vs]
  VI measurement/2(Is) -> [Is]
  Qset/1 -> VSC Control/5(Qset)
  [Vs] -> VSC Control/2(Vabc)
  Edc/1 -> VSC Control/6(Edc)
  connections:
  Three-Phase Transformer (Two Windings)/LConn3 -- Three-Phase Breaker/LConn3
  Three-Phase Transformer (Two Windings)/LConn2 -- Three-Phase Breaker/LConn2
  Three-Phase Transformer (Two Windings)/LConn1 -- Three-Phase Breaker/LConn1
  Three-Phase Transformer (Two Windings)/RConn3 -- VSC Model/LConn3
  Three-Phase Transformer (Two Windings)/RConn2 -- VSC Model/LConn2
  Three-Phase Transformer (Two Windings)/RConn1 -- VSC Model/LConn1
  VI measurement/RConn1 -- A/RConn1
  VI measurement/RConn2 -- B/RConn1
  VI measurement/RConn3 -- C/RConn1
  VI measurement/LConn1 -- Three-Phase Breaker/RConn1
  VI measurement/LConn2 -- Three-Phase Breaker/RConn2
  VI measurement/LConn3 -- Three-Phase Breaker/RConn3

== system Scenario_3_v2/Measurements Phasor/Subsystem1 ==
  abc : Inport
  Gain1 : Gain  Gain=[1 a a2]  SaturateOnIntegerOverflow=on  OutDataTypeStr=Inherit: Same as input  ParamDataTypeStr=Inherit: Same as input
  Gain3 : Gain  Gain=1/3  SaturateOnIntegerOverflow=on  OutDataTypeStr=Inherit: Same as input  ParamDataTypeStr=Inherit: Same as input
  Sum : Sum  Inputs=1  InputSameDT=on  SaturateOnIntegerOverflow=on  OutDataTypeStr=Inherit: Same as first input
  seq+ : Outport
  wires:
  Sum/1 -> Gain3/1
  abc/1 -> Gain1/1
  Gain1/1 -> Sum/1
  Gain3/1 -> seq+/1

== system Scenario_3_v2/Measurements Phasor/Subsystem10 ==
  abc : Inport
  Gain1 : Gain  Gain=[1 a a2]  SaturateOnIntegerOverflow=on  OutDataTypeStr=Inherit: Same as input  ParamDataTypeStr=Inherit: Same as input
  Gain3 : Gain  Gain=1/3  SaturateOnIntegerOverflow=on  OutDataTypeStr=Inherit: Same as input  ParamDataTypeStr=Inherit: Same as input
  Sum : Sum  Inputs=1  InputSameDT=on  SaturateOnIntegerOverflow=on  OutDataTypeStr=Inherit: Same as first input
  seq+ : Outport
  wires:
  Sum/1 -> Gain3/1
  abc/1 -> Gain1/1
  Gain1/1 -> Sum/1
  Gain3/1 -> seq+/1

== system Scenario_3_v2/Measurements Phasor/Subsystem11 ==
  abc : Inport
  Gain1 : Gain  Gain=[1 a a2]  SaturateOnIntegerOverflow=on  OutDataTypeStr=Inherit: Same as input  ParamDataTypeStr=Inherit: Same as input
  Gain3 : Gain  Gain=1/3  SaturateOnIntegerOverflow=on  OutDataTypeStr=Inherit: Same as input  ParamDataTypeStr=Inherit: Same as input
  Sum : Sum  Inputs=1  InputSameDT=on  SaturateOnIntegerOverflow=on  OutDataTypeStr=Inherit: Same as first input
  seq+ : Outport
  wires:
  Sum/1 -> Gain3/1
  abc/1 -> Gain1/1
  Gain1/1 -> Sum/1
  Gain3/1 -> seq+/1

== system Scenario_3_v2/Measurements Phasor/Subsystem12 ==
  abc : Inport
  Gain1 : Gain  Gain=[1 a a2]  SaturateOnIntegerOverflow=on  OutDataTypeStr=Inherit: Same as input  ParamDataTypeStr=Inherit: Same as input
  Gain3 : Gain  Gain=1/3  SaturateOnIntegerOverflow=on  OutDataTypeStr=Inherit: Same as input  ParamDataTypeStr=Inherit: Same as input
  Sum : Sum  Inputs=1  InputSameDT=on  SaturateOnIntegerOverflow=on  OutDataTypeStr=Inherit: Same as first input
  seq+ : Outport
  wires:
  Sum/1 -> Gain3/1
  abc/1 -> Gain1/1
  Gain1/1 -> Sum/1
  Gain3/1 -> seq+/1

== system Scenario_3_v2/Measurements Phasor/Subsystem13 ==
  abc : Inport
  Gain1 : Gain  Gain=[1 a a2]  SaturateOnIntegerOverflow=on  OutDataTypeStr=Inherit: Same as input  ParamDataTypeStr=Inherit: Same as input
  Gain3 : Gain  Gain=1/3  SaturateOnIntegerOverflow=on  OutDataTypeStr=Inherit: Same as input  ParamDataTypeStr=Inherit: Same as input
  Sum : Sum  Inputs=1  InputSameDT=on  SaturateOnIntegerOverflow=on  OutDataTypeStr=Inherit: Same as first input
  seq+ : Outport
  wires:
  Sum/1 -> Gain3/1
  abc/1 -> Gain1/1
  Gain1/1 -> Sum/1
  Gain3/1 -> seq+/1

== system Scenario_3_v2/Measurements Phasor/Subsystem2 ==
  abc : Inport
  Gain1 : Gain  Gain=[1 a a2]  SaturateOnIntegerOverflow=on  OutDataTypeStr=Inherit: Same as input  ParamDataTypeStr=Inherit: Same as input
  Gain3 : Gain  Gain=1/3  SaturateOnIntegerOverflow=on  OutDataTypeStr=Inherit: Same as input  ParamDataTypeStr=Inherit: Same as input
  Sum : Sum  Inputs=1  InputSameDT=on  SaturateOnIntegerOverflow=on  OutDataTypeStr=Inherit: Same as first input
  seq+ : Outport
  wires:
  Gain3/1 -> seq+/1
  Gain1/1 -> Sum/1
  abc/1 -> Gain1/1
  Sum/1 -> Gain3/1

== system Scenario_3_v2/Measurements Phasor/Subsystem3 ==
  abc : Inport
  Gain1 : Gain  Gain=[1 a a2]  SaturateOnIntegerOverflow=on  OutDataTypeStr=Inherit: Same as input  ParamDataTypeStr=Inherit: Same as input
  Gain3 : Gain  Gain=1/3  SaturateOnIntegerOverflow=on  OutDataTypeStr=Inherit: Same as input  ParamDataTypeStr=Inherit: Same as input
  Sum : Sum  Inputs=1  InputSameDT=on  SaturateOnIntegerOverflow=on  OutDataTypeStr=Inherit: Same as first input
  seq+ : Outport
  wires:
  Gain3/1 -> seq+/1
  Gain1/1 -> Sum/1
  abc/1 -> Gain1/1
  Sum/1 -> Gain3/1

== system Scenario_3_v2/Measurements Phasor/Subsystem4 ==
  abc : Inport
  Gain1 : Gain  Gain=[1 a a2]  SaturateOnIntegerOverflow=on  OutDataTypeStr=Inherit: Same as input  ParamDataTypeStr=Inherit: Same as input
  Gain3 : Gain  Gain=1/3  SaturateOnIntegerOverflow=on  OutDataTypeStr=Inherit: Same as input  ParamDataTypeStr=Inherit: Same as input
  Sum : Sum  Inputs=1  InputSameDT=on  SaturateOnIntegerOverflow=on  OutDataTypeStr=Inherit: Same as first input
  seq+ : Outport
  wires:
  Sum/1 -> Gain3/1
  abc/1 -> Gain1/1
  Gain1/1 -> Sum/1
  Gain3/1 -> seq+/1

== system Scenario_3_v2/Measurements Phasor/Subsystem5 ==
  abc : Inport
  Gain1 : Gain  Gain=[1 a a2]  SaturateOnIntegerOverflow=on  OutDataTypeStr=Inherit: Same as input  ParamDataTypeStr=Inherit: Same as input
  Gain3 : Gain  Gain=1/3  SaturateOnIntegerOverflow=on  OutDataTypeStr=Inherit: Same as input  ParamDataTypeStr=Inherit: Same as input
  Sum : Sum  Inputs=1  InputSameDT=on  SaturateOnIntegerOverflow=on  OutDataTypeStr=Inherit: Same as first input
  seq+ : Outport
  wires:
  Gain3/1 -> seq+/1
  Gain1/1 -> Sum/1
  abc/1 -> Gain1/1
  Sum/1 -> Gain3/1

== system Scenario_3_v2/Measurements Phasor/Subsystem6 ==
  abc : Inport
  Gain1 : Gain  Gain=[1 a a2]  SaturateOnIntegerOverflow=on  OutDataTypeStr=Inherit: Same as input  ParamDataTypeStr=Inherit: Same as input
  Gain3 : Gain  Gain=1/3  SaturateOnIntegerOverflow=on  OutDataTypeStr=Inherit: Same as input  ParamDataTypeStr=Inherit: Same as input
  Sum : Sum  Inputs=1  InputSameDT=on  SaturateOnIntegerOverflow=on  OutDataTypeStr=Inherit: Same as first input
  seq+ : Outport
  wires:
  Sum/1 -> Gain3/1
  abc/1 -> Gain1/1
  Gain1/1 -> Sum/1
  Gain3/1 -> seq+/1

== system Scenario_3_v2/Measurements Phasor/Subsystem7 ==
  abc : Inport
  Gain1 : Gain  Gain=[1 a a2]  SaturateOnIntegerOverflow=on  OutDataTypeStr=Inherit: Same as input  ParamDataTypeStr=Inherit: Same as input
  Gain3 : Gain  Gain=1/3  SaturateOnIntegerOverflow=on  OutDataTypeStr=Inherit: Same as input  ParamDataTypeStr=Inherit: Same as input
  Sum : Sum  Inputs=1  InputSameDT=on  SaturateOnIntegerOverflow=on  OutDataTypeStr=Inherit: Same as first input
  seq+ : Outport
  wires:
  Sum/1 -> Gain3/1
  abc/1 -> Gain1/1
  Gain1/1 -> Sum/1
  Gain3/1 -> seq+/1

== system Scenario_3_v2/Measurements Phasor/Subsystem8 ==
  abc : Inport
  Gain1 : Gain  Gain=[1 a a2]  SaturateOnIntegerOverflow=on  OutDataTypeStr=Inherit: Same as input  ParamDataTypeStr=Inherit: Same as input
  Gain3 : Gain  Gain=1/3  SaturateOnIntegerOverflow=on  OutDataTypeStr=Inherit: Same as input  ParamDataTypeStr=Inherit: Same as input
  Sum : Sum  Inputs=1  InputSameDT=on  SaturateOnIntegerOverflow=on  OutDataTypeStr=Inherit: Same as first input
  seq+ : Outport
  wires:
  Sum/1 -> Gain3/1
  abc/1 -> Gain1/1
  Gain1/1 -> Sum/1
  Gain3/1 -> seq+/1

== system Scenario_3_v2/Measurements Phasor/Subsystem9 ==
  abc : Inport
  Gain1 : Gain  Gain=[1 a a2]  SaturateOnIntegerOverflow=on  OutDataTypeStr=Inherit: Same as input  ParamDataTypeStr=Inherit: Same as input
  Gain3 : Gain  Gain=1/3  SaturateOnIntegerOverflow=on  OutDataTypeStr=Inherit: Same as input  ParamDataTypeStr=Inherit: Same as input
  Sum : Sum  Inputs=1  InputSameDT=on  SaturateOnIntegerOverflow=on  OutDataTypeStr=Inherit: Same as first input
  seq+ : Outport
  wires:
  Sum/1 -> Gain3/1
  abc/1 -> Gain1/1
  Gain1/1 -> Sum/1
  Gain3/1 -> seq+/1

== system Scenario_3_v2/AC network/Exciter System/PSS1 ==
  note: Power System Stabilizer (PSS2A)
  dw : Inport
  Pgen : Inport  Port=2
  Gain : Gain  Gain=Ks1
  Gain1 : Gain  Gain=Ks3
  Saturation : Saturate  UpperLimit=Vstmax  LowerLimit=Vstmin
  Sum1 : Sum  Inputs=|++
  Sum2 : Sum  Inputs=|+-
  Transfer Fcn1 : TransferFcn  Numerator=[Tw1 0]  Denominator=[Tw1 1]
  Transfer Fcn2 : TransferFcn  Numerator=[Tw3 0]  Denominator=[Tw3 1]
  Transfer Fcn3 : TransferFcn  Numerator=[Tw2 0]  Denominator=[Tw2 1]
  Transfer Fcn4 : TransferFcn  Denominator=[T6 1]
  Transfer Fcn5 : TransferFcn  Numerator=[T8 1].^N  Denominator=[T9 1].^(M*N)
  Transfer Fcn6 : TransferFcn  Numerator=[T1 1]  Denominator=[T2 1]
  Transfer Fcn7 : TransferFcn  Numerator=[T3 1]  Denominator=[T4 1]
  Transfer Fcn8 : TransferFcn  Numerator=[Tw4 0]  Denominator=[Tw4 1]
  Transfer Fcn9 : TransferFcn  Numerator=[Ks2]  Denominator=[T7 1]
  Vothsg : Outport
  wires:
  dw/1 -> Transfer Fcn1/1
  Transfer Fcn1/1 -> Transfer Fcn3/1
  Transfer Fcn3/1 -> Transfer Fcn4/1
  Transfer Fcn4/1 -> Sum1/1
  Sum1/1 -> Transfer Fcn5/1
  Transfer Fcn5/1 -> Sum2/1
  Sum2/1 -> Gain/1
  Gain/1 -> Transfer Fcn6/1
  Transfer Fcn6/1 -> Transfer Fcn7/1
  Transfer Fcn7/1 -> Saturation/1
  Saturation/1 -> Vothsg/1
  Pgen/1 -> Transfer Fcn2/1
  Transfer Fcn2/1 -> Transfer Fcn8/1
  Transfer Fcn8/1 -> Transfer Fcn9/1
  Gain1/1 -> Sum1/2
  Transfer Fcn9/1 -> Gain1/1, Sum2/2

== system Scenario_3_v2/AC network/Exciter System/PSS1 backup ==
  note: Power System Stabilizer (PSS2A)
  dw : Inport
  Pgen : Inport  Port=2
  Gain : Gain  Gain=Ks1
  Gain1 : Gain  Gain=Ks3
  Saturation : Saturate  UpperLimit=Vstmax  LowerLimit=Vstmin
  Sum1 : Sum  Inputs=|++
  Sum2 : Sum  Inputs=|+-
  Transfer Fcn1 : TransferFcn  Numerator=[Tw1 0]  Denominator=[Tw1 1]
  Transfer Fcn2 : TransferFcn  Numerator=[Tw3 0]  Denominator=[Tw3 1]
  Transfer Fcn3 : TransferFcn  Numerator=[Tw2 0]  Denominator=[Tw2 1]
  Transfer Fcn4 : TransferFcn  Denominator=[T6 1]
  Transfer Fcn5 : TransferFcn  Numerator=[T8 1].^N  Denominator=[T9 1].^(M*N)
  Transfer Fcn6 : TransferFcn  Numerator=[T1 1]  Denominator=[T2 1]
  Transfer Fcn7 : TransferFcn  Numerator=[T3 1]  Denominator=[T4 1]
  Transfer Fcn8 : TransferFcn  Numerator=[Tw4 0]  Denominator=[Tw4 1]
  Transfer Fcn9 : TransferFcn  Numerator=[Ks2]  Denominator=[T7 1]
  Vothsg : Outport
  wires:
  Transfer Fcn9/1 -> Sum2/2, Gain1/1
  Gain1/1 -> Sum1/2
  Transfer Fcn8/1 -> Transfer Fcn9/1
  Transfer Fcn2/1 -> Transfer Fcn8/1
  Pgen/1 -> Transfer Fcn2/1
  Saturation/1 -> Vothsg/1
  Transfer Fcn7/1 -> Saturation/1
  Transfer Fcn6/1 -> Transfer Fcn7/1
  Gain/1 -> Transfer Fcn6/1
  Sum2/1 -> Gain/1
  Transfer Fcn5/1 -> Sum2/1
  Sum1/1 -> Transfer Fcn5/1
  Transfer Fcn4/1 -> Sum1/1
  Transfer Fcn3/1 -> Transfer Fcn4/1
  Transfer Fcn1/1 -> Transfer Fcn3/1
  dw/1 -> Transfer Fcn1/1

== system Scenario_3_v2/AC network/Exciter System/SEXS ==
  note: The controller parameters provided by ENTSO-E
      | define different names for the parameters:
      |
      | ENTSO-E = IEEE Std 421.5-2005
      | Ta = Tc
      | Tb = Tb
      | K = Ka
      | Te = Ta
      | Emax = Vrmax
      | Emin = Vrmin
  note: The exciter model provided by ENTSO-E most similar to the IEEE is the Type AC4A excitation system model
  Vref : Inport
  Vc : Inport  Port=2
  Vs : Inport  Port=3
  1st ord transfer fcn windup limiter : Subsystem  mask{Gain=K, tau=Te, Vmax=Emax, Vmin=Emin, y0=Vf0}
      mask prompts: tau "Time constant"; y0 "Initial output"
  Constant : Constant  Value=Vf0/K
  Saturation : Saturate  Commented=through  UpperLimit=0.1  LowerLimit=-0.1
  Sum : Sum  Inputs=+-+
  Sum1 : Sum  Inputs=|++
  Transfer Fcn (with initial outputs)1 : simulink_extras/Additional Linear/Transfer Fcn (with initial outputs)  N=[Ta 1]  D=[Tb 1]  Y0=Vf0/K  U0=Vf0/K
  Efd : Outport
  wires:
  1st ord transfer fcn windup limiter/1(Out1) -> Efd/1
  Vs/1 -> Sum/3
  Vref/1 -> Sum/1
  Vc/1 -> Sum/2
  Transfer Fcn (with initial outputs)1/1 -> 1st ord transfer fcn windup limiter/1(In1)
  Saturation/1 -> Transfer Fcn (with initial outputs)1/1
  Sum/1 -> Sum1/1
  Sum1/1 -> Saturation/1
  Constant/1 -> Sum1/2

== system Scenario_3_v2/AC network/Exciter System/TR and LC_test ==
  note: Terminal voltage transducer and optional load compensation
  note: compensated
      | impedance
  note: Vt and It should be phasors (complex quantities)
  note: Fig 4.1 of IEEE Std 421.5-2005
  note: Rc and Xc should be negative values in case of voltage regulated after an impedance
  Vt : Inport
  It : Inport  Port=2
  Abs : Abs
  Abs1 : Abs
  Rc+jXc : Gain  Gain=abs(Rc+1i*Xc)
  Saturation : Saturate  UpperLimit=1.2  LowerLimit=0.8
  Sum : Sum  Inputs=|+-
  Transfer Fcn (with initial outputs) : simulink_extras/Additional Linear/Transfer Fcn (with initial outputs)  Commented=through  N=[1]  D=[Tr 1]  Y0=1  U0=1
  Vc : Outport
  wires:
  Saturation/1 -> Vc/1
  Vt/1 -> Abs/1
  Transfer Fcn (with initial outputs)/1 -> Saturation/1
  Rc+jXc/1 -> Sum/2
  Sum/1 -> Transfer Fcn (with initial outputs)/1
  It/1 -> Abs1/1
  Abs/1 -> Sum/1
  Abs1/1 -> Rc+jXc/1

== system Scenario_3_v2/G1/VSC v2/VI measurement ==
  Current Measurement : powerlib/Measurements/Current Measurement  PhasorSimulation=off  OutputType=Complex  PSBequivalent=0
  Current Measurement1 : powerlib/Measurements/Current Measurement  PhasorSimulation=off  OutputType=Complex  PSBequivalent=0
  Current Measurement2 : powerlib/Measurements/Current Measurement  PhasorSimulation=off  OutputType=Complex  PSBequivalent=0
  Ground : powerlib/Elements/Ground  LConnTagsString=a
  Ground1 : powerlib/Elements/Ground  LConnTagsString=a
  Ground2 : powerlib/Elements/Ground  LConnTagsString=a
  Mux : Mux  Inputs=3
  Mux1 : Mux  Inputs=3
  Voltage Measurement : powerlib/Measurements/Voltage Measurement  PhasorSimulation=off  OutputType=Complex  PSBequivalent=0
  Voltage Measurement1 : powerlib/Measurements/Voltage Measurement  PhasorSimulation=off  OutputType=Complex  PSBequivalent=0
  Voltage Measurement2 : powerlib/Measurements/Voltage Measurement  PhasorSimulation=off  OutputType=Complex  PSBequivalent=0
  A : PMIOPort  Side=Left
  B : PMIOPort  Port=2  Side=Left
  C : PMIOPort  Port=3  Side=Left
  a : PMIOPort  Port=4  Side=Right
  b : PMIOPort  Port=5  Side=Right
  c : PMIOPort  Port=6  Side=Right
  Vs : Outport
  Is : Outport  Port=2
  wires:
  Mux1/1 -> Is/1
  Mux/1 -> Vs/1
  Voltage Measurement1/1 -> Mux/2
  Voltage Measurement2/1 -> Mux/3
  Current Measurement2/1 -> Mux1/3
  Voltage Measurement/1 -> Mux/1
  Current Measurement/1 -> Mux1/1
  Current Measurement1/1 -> Mux1/2
  connections:
  Voltage Measurement/LConn1 -- Current Measurement/LConn1 -- A/RConn1
  Current Measurement2/LConn1 -- Voltage Measurement2/LConn1 -- C/RConn1
  Current Measurement1/LConn1 -- Voltage Measurement1/LConn1 -- B/RConn1
  Current Measurement1/RConn1 -- b/RConn1
  Current Measurement/RConn1 -- a/RConn1
  Ground/LConn1 -- Voltage Measurement/LConn2
  Current Measurement2/RConn1 -- c/RConn1
  Ground1/LConn1 -- Voltage Measurement1/LConn2
  Ground2/LConn1 -- Voltage Measurement2/LConn2
